simulink model "liqlevel_exch01"  (Simulink 10.2)
settings: Solver=ode45  StartTime=0.0  StopTime=(length(uin)-1)*Ts  RelTol=1e-3  EnableMultiTasking=on
model workspace (MATLAB code in the model file):
  | Cv = 1.5; Ac = 2;
  | x0 = 9;
  | uss = Cv*sqrt(x0);
  | 
  | tau = Ac*2*sqrt(x0)/Cv;
  | sampfact = 8;
  | Ts = tau/sampfact;
  | f_max = (4/sampfact)/(2*pi);
  | B_max = 1/5;
  | 
  | usig = idinput(2555,'prbs',[0 B_max],[-1 1]);
  | uin = [(0:1:length(usig)-1)'*Ts (usig*0.05+1)*uss];
settings Model: Creator=arun  LastModifiedBy=Monish Kumar  ExtModeAutoUpdateStatusClock=off
settings DataIOCC: SaveState=on
settings OptimizationCC: ExpressionDepthLimit=2147483647  InitFltsAndDblsToZero=on
settings DebuggingCC: SaveWithParameterizedLinksMsg=none  SolverPrmCheckMsg=warning  StateNameClashWarn=warning
settings GRTTargetCC: TargetFcnLib=ansi_tfl_tmw.mat

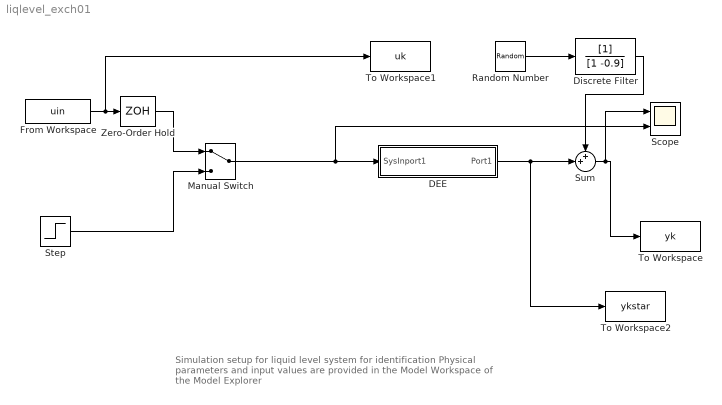
== system liqlevel_exch01 ==
  note: Simulation setup for liquid level system for identification
      |
      | Physical parameters and input values are provided
      | in the Model Workspace of the Model Explorer
  DEE : Subsystem  mask(Differential Equation Editor (DEE)){}
      settings: OpenFcn=diffeqed
      mask Display: disp('Differential Equation\n Editor')
  Discrete Filter : DiscreteFilter  Denominator=[1 -0.9]
  From Workspace : FromWorkspace  VariableName=uin  SampleTime=Ts  Interpolate=off  OutputAfterFinalValue=Holding final value
  Manual Switch : ManualSwitch
  Random Number : RandomNumber  Variance=0.02092  SampleTime=Ts
  Scope : Scope  NumInputPorts=2
  Step : Step  Time=5  Before=uss  After=1.05*uss  SampleTime=0
  Sum : Sum  Inputs=++|
  To Workspace : ToWorkspace  VariableName=yk  SampleTime=Ts
  To Workspace1 : ToWorkspace  VariableName=uk  SampleTime=Ts
  To Workspace2 : ToWorkspace  VariableName=ykstar  SampleTime=Ts
  Zero-Order Hold : ZeroOrderHold  SampleTime=Ts
  wires:
  Manual Switch/1 -> Scope/2, DEE/1(SysInport1)
  From Workspace/1 -> Zero-Order Hold/1, To Workspace1/1
  Step/1 -> Manual Switch/2
  Zero-Order Hold/1 -> Manual Switch/1
  DEE/1(Port1) -> Sum/2, To Workspace2/1
  Random Number/1 -> Discrete Filter/1
  Sum/1 -> To Workspace/1, Scope/1
  Discrete Filter/1 -> Sum/1

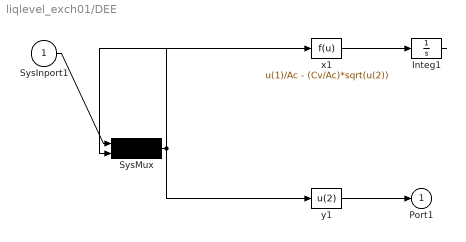
== system liqlevel_exch01/DEE ==
  SysInport1 : Inport
  Integ1 : Integrator  InitialCondition=x0
  SysMux : Mux  Inputs=2
  x1 : Fcn  Expr=u(1)/Ac - (Cv/Ac)*sqrt(u(2))
  y1 : Fcn  Expr=u(2)
  Port1 : Outport
  wires:
  SysInport1/1 -> SysMux/1
  SysMux/1 -> x1/1, y1/1
  x1/1 -> Integ1/1
  Integ1/1 -> SysMux/2
  y1/1 -> Port1/1
